simulink model "density_model"  (R2016a)
settings: Solver=VariableStepAuto  StartTime=0.0  StopTime=10.0  RelTol=1e-3
values from neighbouring files (symbols this model uses):
  rho0 = 1.225    [Simulink_Constants.m]
settings Model: Creator=Bakry  LastModifiedBy=Bakry

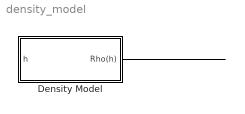
== system density_model ==
  Density Model : Subsystem
  wires:
  ? -> Density Model/1(h)
  Density Model/1(Rho(h)) -> ?

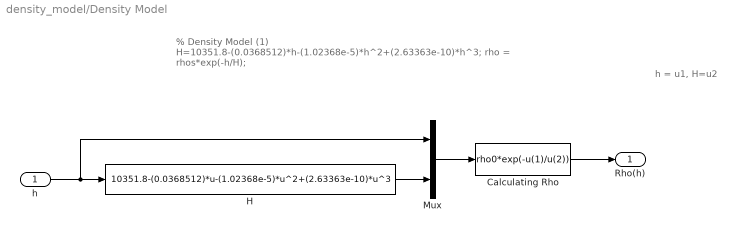
== system density_model/Density Model ==
  note: h = u1, H=u2
  note: % Density Model (1)
      | H=10351.8-(0.0368512)*h-(1.02368e-5)*h^2+(2.63363e-10)*h^3;
      | rho = rhos*exp(-h/H);
  h : Inport
  Calculating Rho : Fcn  Expr=rho0*exp(-u(1)/u(2))
  H : Fcn  Expr=10351.8-(0.0368512)*u-(1.02368e-5)*u^2+(2.63363e-10)*u^3
  Mux : Mux  Inputs=2
  Rho(h) : Outport
  wires:
  h/1 -> Mux/1, H/1
  H/1 -> Mux/2
  Mux/1 -> Calculating Rho/1
  Calculating Rho/1 -> Rho(h)/1
